simulink subsystem "Vehicle1DBasicRefSub"  (R2020a)
settings: Solver=VariableStepAuto  StartTime=0.0  StopTime=10.0  RelTol=1e-3
libraries: nesl_utility x4
settings Model: Creator=isaacito  LastModifiedBy=isaacito

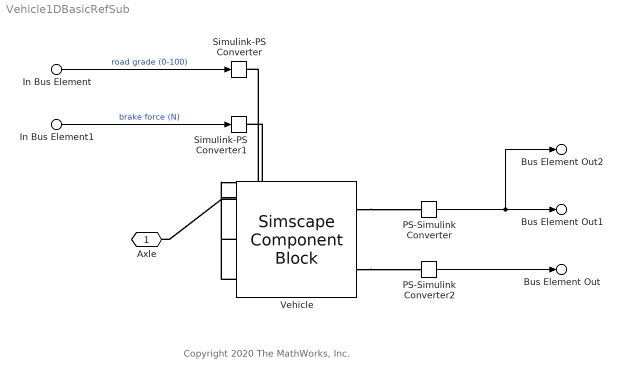
== system Vehicle1DBasicRefSub ==
  note: Copyright 2020 The MathWorks, Inc.
  In Bus Element : Inport  PortName=DrvEnv  Element=RoadGrade
      settings: AttributesFormatString=%<Unit>
  In Bus Element1 : Inport  PortName=DrvEnv  Element=BrakeForce
      settings: AttributesFormatString=%<Unit>
  PS-Simulink Converter : nesl_utility/PS-Simulink Converter  PhysicalDomain=network_engine_domain  SubClassName=ps_output  LeftPortType=input  RightPortType=output  PseudoPeriodic=off  Frequencies=[]  Unit=km/hr  AffineConversion=off
  PS-Simulink Converter2 : nesl_utility/PS-Simulink Converter  PhysicalDomain=network_engine_domain  SubClassName=ps_output  LeftPortType=input  RightPortType=output  PseudoPeriodic=off  Frequencies=[]  Unit=1  AffineConversion=off
  Simulink-PS Converter : nesl_utility/Simulink-PS Converter  PhysicalDomain=network_engine_domain  SubClassName=ps_input  LeftPortType=input  RightPortType=output  PseudoPeriodic=off  Frequencies=[]  NoiseDistribution=none  NoiseParameters=[]  Unit=1  AffineConversion=off  FilteringAndDerivatives=provide  SimscapeFilterOrder=1  InputFilterTimeConstant=0.001  UdotUserProvided=0
  Simulink-PS Converter1 : nesl_utility/Simulink-PS Converter  PhysicalDomain=network_engine_domain  SubClassName=ps_input  LeftPortType=input  RightPortType=output  PseudoPeriodic=off  Frequencies=[]  NoiseDistribution=none  NoiseParameters=[]  Unit=N  AffineConversion=off  FilteringAndDerivatives=provide  SimscapeFilterOrder=1  InputFilterTimeConstant=0.001  UdotUserProvided=0
  Vehicle : SimscapeComponentBlock  SourceFile=Vehicle1DBasic  ComponentPath=Vehicle1DBasic  ComponentVariants="[\"Vehicle1DBasic\"]"  ComponentVariantNames="[\"Vehicle1DBasic\"]"  ClassName=Vehicle1DBasic  SchemaVersion=1  M_e=vehicle.vehMass_kg kg  R_tire=vehicle.tireRollingRadius_cm cm  A_rl=vehicle.roadLoadA_N N  B_rl=vehicle.roadLoadB_N_per_kph N*hr/km  C_rl=vehicle.roadLoadC_N_per_kph2 N*hr^2/km^2  ShowBrakeIn=simscape.enum.onoff.on  ShowGradeIn=simscape.enum.onoff.on  grav=9.81 m/s^2  ShowVelOut=simscape.enum.onoff.on  ShowGOut=simscape.enum.onoff.on  v_specify=off  v_priority=High  v=0 km/hr  v_nominal_specify=off  v_nominal_unit=km/hr  v_nominal_value=1
      settings: CopyFcn=simscape.engine.sli.internal.componentblockcallback(gcbh,'COPY')  PreCopyFcn=simscape.engine.sli.internal.componentblockcallback(gcbh,'PRECOPY')  PreDeleteFcn=simscape.engine.sli.internal.componentblockcallback(gcbh,'PREDELETE')  InternalSimscapePortConfiguration="{\"Bottom\":[],\"Left\":[{\"id\":\"Axle\",\"label\":\"Axle\",\"type\":\"foundation.mechanical.rotational.rotational\"}],\"Right\":[{\"id\":\"v_out\",\"label\":\"V\",\"type\":\"output\"},{\"id\":\"G\",\"label\":\"G\",\"type\":\"output\"}],\"Top\":[{\"id\":\"brkF\",\"label\":\"Brake\",\"type\":\"input\"},{\"id\":\"grade_pct\",\"label\":\"Grade\",\"type\":\"input\"}]}"
      mask Type: Vehicle 1D Basic
  Axle : PMIOPort  Side=Left
  Bus Element Out : Outport  PortName=Info  Element=G
      settings: AttributesFormatString=%<Unit>
  Bus Element Out1 : Outport  PortName=Info  Element=VehSpd
      settings: AttributesFormatString=%<Unit>
  Bus Element Out2 : Outport  Port=2  PortName=Sensor  Element=VehSpd
      settings: AttributesFormatString=%<Unit>
  wires:
  PS-Simulink Converter/1 -> Bus Element Out1/1, Bus Element Out2/1
  PS-Simulink Converter2/1 -> Bus Element Out/1
  In Bus Element/1 -> Simulink-PS Converter/1  "road grade (0-100)"
  In Bus Element1/1 -> Simulink-PS Converter1/1  "brake force (N)"
  connections:
  Vehicle/RConn2 -- PS-Simulink Converter2/LConn1
  Vehicle/RConn1 -- PS-Simulink Converter/LConn1
  Vehicle/LConn1 -- Axle/RConn1
  Vehicle/LConn3 -- Simulink-PS Converter/RConn1
  Vehicle/LConn2 -- Simulink-PS Converter1/RConn1
